simulink model "ICCMA_posicast_23_parallelGCNM_FO"  (R2022b)
settings: Solver=FixedStepAuto  StartTime=0.0  StopTime=1  FixedStep=1e-6  RelTol=1e-3
values from neighbouring files (symbols this model uses):
  alphaFoPar = alpha    [Flyback_SOC_benchmark_Start_parallel.m]
  amp = 1    [Flyback_SOC_benchmark_Start_parallel.m]
  delta = 0.7    [Flyback_SOC_benchmark_Start_parallel.m]
  k1 = 7.51277596604741e-09    (= 7.51277596605e-09)    [Flyback_SOC_benchmark_Start_parallel.m]
  k2 = 1e5    (= 100000)    [Flyback_SOC_benchmark_Start_parallel.m]
  maxKd = 0.1    [Flyback_SOC_benchmark_Start_parallel.m]
  maxKi = 8e5    (= 800000)    [Flyback_SOC_benchmark_Start_parallel.m]
  maxKp = 1e-3    (= 0.001)    [Flyback_SOC_benchmark_Start_parallel.m]
  maxLimDelta = 1.1    [Flyback_SOC_benchmark_Start_parallel.m]
  maxLimTd = 1e-5    (= 1e-05)    [Flyback_SOC_benchmark_Start_parallel.m]
  minKd = 0.001    [Flyback_SOC_benchmark_Start_parallel.m]
  minKi = 8e4    (= 80000)    [Flyback_SOC_benchmark_Start_parallel.m]
  minKp = 1e-6    (= 1e-06)    [Flyback_SOC_benchmark_Start_parallel.m]
  minLimDelta = 0.9    [Flyback_SOC_benchmark_Start_parallel.m]
  minLimTd = 1e-7    (= 1e-07)    [Flyback_SOC_benchmark_Start_parallel.m]
  N = 100    [Flyback_SOC_benchmark_Start_parallel.m]
  optimPeriod = 1/1000    (= 0.001)    [Flyback_SOC_benchmark_Start_parallel.m]
  OVLim = 1    [Flyback_SOC_benchmark_Start_parallel.m]
  refSignalPeriod = 1/1000    (= 0.001)    [Flyback_SOC_benchmark_Start_parallel.m]
  resetThreshold = 0.1    [Flyback_SOC_benchmark_Start_parallel.m]
  td = 24e-6    (= 2.4e-05)    [Flyback_SOC_benchmark_Start_parallel.m]
  TSLim = 65    [Flyback_SOC_benchmark_Start_parallel.m]
libraries: cstblocks x28, dspmathops x7, slpidlib x7
(part 1 of 2)
settings Model: Creator=justu  LastModifiedBy=jairo
settings ModelReferenceCC: EnableRefExpFcnMdlSchedulingChecks=on

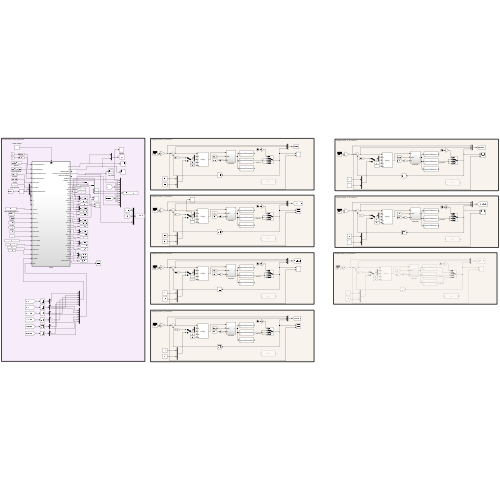
[thumbnail: Simulink's stored preview of the top-level diagram]
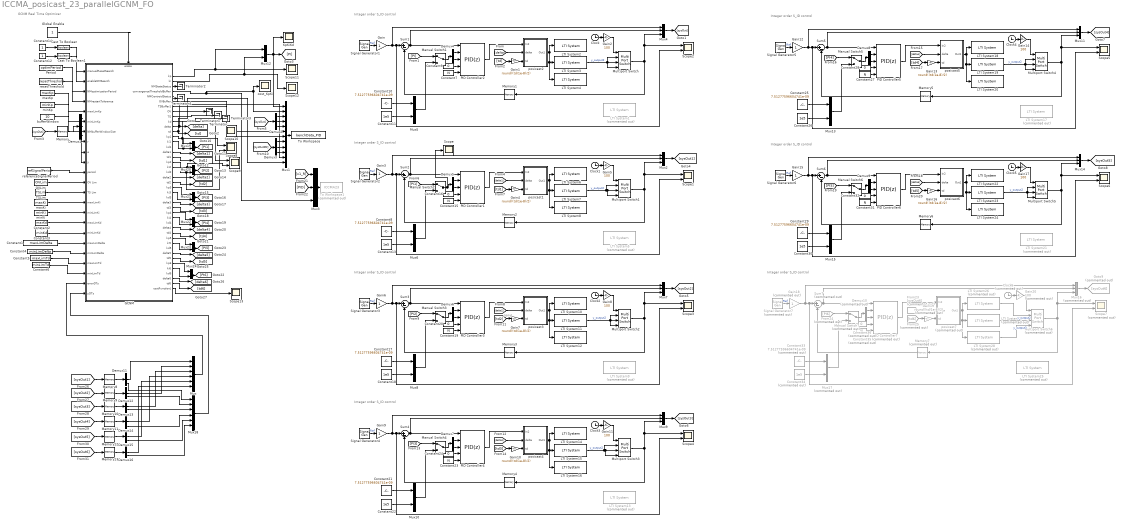
== system ICCMA_posicast_23_parallelGCNM_FO ==
  note: convJ
  note: GCNM Real Time Optimizer
  note: Integer order S_ID control
  note: Integer order S_ID control
  note: Integer order S_ID control
  note: Integer order S_ID control
  note: Integer order S_ID control
  note: Integer order S_ID control
  note: Integer order S_ID control
  Cast To Boolean : DataTypeConversion  OutDataTypeStr=boolean  SaturateOnIntegerOverflow=off  RndMeth=Floor
  Cast To Boolean1 : DataTypeConversion  OutDataTypeStr=boolean  SaturateOnIntegerOverflow=off  RndMeth=Floor
  Clock{,1..5} (6 alike) : Clock
  Clock6 : Clock  Commented=on
  Constant1 : Constant  Value=maxLimDelta
  Constant{8,10,17,21,25,29} (6 alike) : Constant  Value=7.51277596604741e-09
  Constant{11,13,18,22,26,30} (6 alike) : Constant  Value=1e5
  Constant12 : Constant  OutDataTypeStr=boolean
  Constant14 : Constant
  Constant{7,15,19,23,27,31} (6 alike) : Constant  Value=N
  Constant{9,16,20,24,28,32} (6 alike) : Constant  Value=0
  Constant2 : Constant  Value=maxKd
  Constant3 : Constant  Value=minKd
  Constant33 : Constant  Commented=on  Value=7.51277596604741e-09
  Constant34 : Constant  Commented=on  Value=1e5
  Constant35 : Constant  Commented=on  Value=N
  Constant36 : Constant  Commented=on  Value=0
  Constant4 : Constant  Value=minLimDelta
  Constant5 : Constant  Value=maxLimTd
  Constant6 : Constant  Value=minLimTd
  Demux{1..3,11..16} (9 alike) : Demux  Outputs=3
  Demux10 : Demux  Commented=on  Outputs=2
  Demux{4..9} (6 alike) : Demux  Outputs=2
  From23 : From  Commented=on  GotoTag=sysOut6
  From24 : From  Commented=on  GotoTag=PI6
  From25 : From  Commented=on  GotoTag=td6
  GCNM : Subsystem
  Gain{,3,6,9,12,15} (6 alike) : Gain
  Gain{1,4,7,10,13,16} (6 alike) : Gain  Gain=round((td/1e-8)/2)
  Gain{2,5,8,11,14,17} (6 alike) : Gain  Gain=100
  Gain18 : Gain  Commented=on
  Gain19 : Gain  Commented=on  Gain=round((td/1e-8)/2)
  Gain20 : Gain  Commented=on  Gain=100
  Global Enable : Constant
  Goto9 : Goto  Commented=on  GotoTag=sysOut6
  KpKiKd : Scope
  LTI System{1,5,9,13,17,21,25} (7 alike) : cstblocks/LTI System  Commented=on  sys=flybackTFDiscrete  IC=[]
  LTI System{2,6,10,14,18,22} (6 alike) : cstblocks/LTI System  sys=flybackTFDiscrete1  IC=[]
  LTI System{3,7,11,15,19,23} (6 alike) : cstblocks/LTI System  sys=flybackTFDiscrete2  IC=[]
  LTI System{4,8,12,16,20,24} (6 alike) : cstblocks/LTI System  sys=flybackTFDiscrete3  IC=[]
  LTI System26 : cstblocks/LTI System  Commented=on  sys=flybackTFDiscrete1  IC=[]
  LTI System27 : cstblocks/LTI System  Commented=on  sys=flybackTFDiscrete2  IC=[]
  LTI System28 : cstblocks/LTI System  Commented=on  sys=flybackTFDiscrete3  IC=[]
  Manual Switch{1..6} (6 alike) : ManualSwitch
  Manual Switch7 : ManualSwitch  Commented=on
  Memory{,8..13} (7 alike) : Memory  InheritSampleTime=on  LinearizeAsDelay=on
  Memory{1..6} (6 alike) : Memory
  Memory7 : Memory  Commented=on
  Multiport Switch{,1..5} (6 alike) : MultiPortSwitch  DataPortOrder=Specify indices  DataPortIndices={5,10,15}  DiagnosticForDefault=None  SaturateOnIntegerOverflow=off  InputSameDT=off
  Multiport Switch6 : MultiPortSwitch  Commented=on  DataPortOrder=Specify indices  DataPortIndices={5,10,15}  DiagnosticForDefault=None  SaturateOnIntegerOverflow=off  InputSameDT=off
  Mux : Mux  Inputs=6
  Mux1 : Mux  Inputs=12
  Mux{5..6,8,10,12..13,15,19..24} (13 alike) : Mux  Inputs=2
  Mux{2..4,7,9,11,14} (7 alike) : Mux  Inputs=3
  Mux16 : Mux  Commented=on  Inputs=3
  Mux17 : Mux  Commented=on  Inputs=2
  Mux18 : Mux  Inputs=6
  OVLim : Constant  Value=OVLim
  PID Controller{1..6} (6 alike) : slpidlib/PID Controller  Controller=PID  Form=Parallel  TimeDomain=Discrete-time  UseExternalTs=off  SampleTime=-1  IntegratorMethod=Forward Euler  FilterMethod=Forward Euler  ControllerParametersSource=external  P=1  I=100  UseKiTs=off  D=0  N=100  UseFilter=on  TunerSelectOption=Transfer Function Based (PID Tuner App)  InitialConditionSource=internal  InitialConditionForIntegrator=0  InitialConditionForFilter=0  DifferentiatorICPrevScaledInput=0  ExternalReset=none  TrackingMode=off  Kt=1  LimitOutput=off  SatLimitsSource=internal  UpperSaturationLimit=inf  LowerSaturationLimit=-inf  LinearizeAsGain=on  AntiWindupMode=none  Kb=1  LimitIntegrator=off  UpperIntegratorSaturationLimit=inf  LowerIntegratorSaturationLimit=-inf  POutMin=[]  POutMax=[]  IOutMin=[]  IOutMax=[]  DOutMin=[]  DOutMax=[]  NOutMin=[]  NOutMax=[]  SumOutMin=[]  SumOutMax=[]  SaturationOutMin=[]  SaturationOutMax=[]  PParamMin=[]  PParamMax=[]  IParamMin=[]  IParamMax=[]  DParamMin=[]  DParamMax=[]  NParamMin=[]  NParamMax=[]  KbParamMin=[]  KbParamMax=[]  KtParamMin=[]  KtParamMax=[]  KbOutMin=[]  KbOutMax=[]  KtOutMin=[]  KtOutMax=[]  IntegratorOutMin=[]  IntegratorOutMax=[]  FilterOutMin=[]  FilterOutMax=[]  SumI1OutMin=[]  SumI1OutMax=[]  SumI2OutMin=[]  SumI2OutMax=[]  SumI3OutMin=[]  SumI3OutMax=[]  SumI4OutMin=[]  SumI4OutMax=[]  SumDOutMin=[]  SumDOutMax=[]  DifferentiatorOutMin=[]  DifferentiatorOutMax=[]  FilterDiffOutCoefMin=[]  FilterDiffOutCoefMax=[]  ReciprocalOutMin=[]  ReciprocalOutMax=[]  SumDenOutMin=[]  SumDenOutMax=[]  SumNumOutMin=[]  SumNumOutMax=[]  DivideOutMin=[]  DivideOutMax=[]  UdiffTsProdOutMin=[]  UdiffTsProdOutMax=[]  NTsProdOutMin=[]  NTsProdOutMax=[]  UintegralTsProdOutMin=[]  UintegralTsProdOutMax=[]  UngainTsProdOutMin=[]  UngainTsProdOutMax=[]  ClampingZeroOutDataTypeStr=Inherit: Inherit via back propagation  ClampingZeroOutMin=[]  ClampingZeroOutMax=[]  FilterDenConstantOutDataTypeStr=Inherit: Inherit via back propagation  FilterDenConstantOutMin=[]  FilterDenConstantOutMax=[]  PCopyOutDataTypeStr=Inherit: Inherit via back propagation  PCopyOutMin=[]  PCopyOutMax=[]  NCopyOutDataTypeStr=Inherit: Inherit via back propagation  NCopyOutMin=[]  NCopyOutMax=[]  IntegratorContinuousStateAttributes=''  IntegratorStateMustResolveToSignalObject=off  IntegratorRTWStateStorageClass=Auto  FilterContinuousStateAttributes=''  FilterStateMustResolveToSignalObject=off  FilterRTWStateStorageClass=Auto  ParallelPVariant=ExternalParameters  IdealPVariant=Disabled  IVariant=ExternalParameters  DVariant=ExternalParameters  IntegratorVariant=Discrete  SatVariant=Disabled  AWVariant=Passthrough  PCopyVariant=Disabled  TRVariant=Disabled  FdbkBlocksVariant=Forward  IdealPFdbkVariant=Disabled  SatFdbkVariant=Disabled  DerivativeFilterVariant=ForwardEulerFilter  NVariant=ExternalParameters  NCopyVariant=Disabled  FilterICVariant=InternalICsFilter  IntegratorICVariant=InternalICs  ExternalResetVariant=Disabled  TRSumVariant=Passthrough  SumFdbkVariant=Disabled  SumVariant=Sum_PID  TsampFilterVariant=InternalTs  TsampNgainVariant=Passthrough  TsampIntegralVariant=Passthrough  ExternalSaturationOutDataTypeStr=Inherit: Same as second input
  PID Controller7 : slpidlib/PID Controller  Commented=on  Controller=PID  Form=Parallel  TimeDomain=Discrete-time  UseExternalTs=off  SampleTime=-1  IntegratorMethod=Forward Euler  FilterMethod=Forward Euler  ControllerParametersSource=external  P=1  I=100  UseKiTs=off  D=0  N=100  UseFilter=on  TunerSelectOption=Transfer Function Based (PID Tuner App)  InitialConditionSource=internal  InitialConditionForIntegrator=0  InitialConditionForFilter=0  DifferentiatorICPrevScaledInput=0  ExternalReset=none  TrackingMode=off  Kt=1  LimitOutput=off  SatLimitsSource=internal  UpperSaturationLimit=inf  LowerSaturationLimit=-inf  LinearizeAsGain=on  AntiWindupMode=none  Kb=1  LimitIntegrator=off  UpperIntegratorSaturationLimit=inf  LowerIntegratorSaturationLimit=-inf  POutMin=[]  POutMax=[]  IOutMin=[]  IOutMax=[]  DOutMin=[]  DOutMax=[]  NOutMin=[]  NOutMax=[]  SumOutMin=[]  SumOutMax=[]  SaturationOutMin=[]  SaturationOutMax=[]  PParamMin=[]  PParamMax=[]  IParamMin=[]  IParamMax=[]  DParamMin=[]  DParamMax=[]  NParamMin=[]  NParamMax=[]  KbParamMin=[]  KbParamMax=[]  KtParamMin=[]  KtParamMax=[]  KbOutMin=[]  KbOutMax=[]  KtOutMin=[]  KtOutMax=[]  IntegratorOutMin=[]  IntegratorOutMax=[]  FilterOutMin=[]  FilterOutMax=[]  SumI1OutMin=[]  SumI1OutMax=[]  SumI2OutMin=[]  SumI2OutMax=[]  SumI3OutMin=[]  SumI3OutMax=[]  SumI4OutMin=[]  SumI4OutMax=[]  SumDOutMin=[]  SumDOutMax=[]  DifferentiatorOutMin=[]  DifferentiatorOutMax=[]  FilterDiffOutCoefMin=[]  FilterDiffOutCoefMax=[]  ReciprocalOutMin=[]  ReciprocalOutMax=[]  SumDenOutMin=[]  SumDenOutMax=[]  SumNumOutMin=[]  SumNumOutMax=[]  DivideOutMin=[]  DivideOutMax=[]  UdiffTsProdOutMin=[]  UdiffTsProdOutMax=[]  NTsProdOutMin=[]  NTsProdOutMax=[]  UintegralTsProdOutMin=[]  UintegralTsProdOutMax=[]  UngainTsProdOutMin=[]  UngainTsProdOutMax=[]  ClampingZeroOutDataTypeStr=Inherit: Inherit via back propagation  ClampingZeroOutMin=[]  ClampingZeroOutMax=[]  FilterDenConstantOutDataTypeStr=Inherit: Inherit via back propagation  FilterDenConstantOutMin=[]  FilterDenConstantOutMax=[]  PCopyOutDataTypeStr=Inherit: Inherit via back propagation  PCopyOutMin=[]  PCopyOutMax=[]  NCopyOutDataTypeStr=Inherit: Inherit via back propagation  NCopyOutMin=[]  NCopyOutMax=[]  IntegratorContinuousStateAttributes=''  IntegratorStateMustResolveToSignalObject=off  IntegratorRTWStateStorageClass=Auto  FilterContinuousStateAttributes=''  FilterStateMustResolveToSignalObject=off  FilterRTWStateStorageClass=Auto  ParallelPVariant=ExternalParameters  IdealPVariant=Disabled  IVariant=ExternalParameters  DVariant=ExternalParameters  IntegratorVariant=Discrete  SatVariant=Disabled  AWVariant=Passthrough  PCopyVariant=Disabled  TRVariant=Disabled  FdbkBlocksVariant=Forward  IdealPFdbkVariant=Disabled  SatFdbkVariant=Disabled  DerivativeFilterVariant=ForwardEulerFilter  NVariant=ExternalParameters  NCopyVariant=Disabled  FilterICVariant=InternalICsFilter  IntegratorICVariant=InternalICs  ExternalResetVariant=Disabled  TRSumVariant=Passthrough  SumFdbkVariant=Disabled  SumVariant=Sum_PID  TsampFilterVariant=InternalTs  TsampNgainVariant=Passthrough  TsampIntegralVariant=Passthrough  ExternalSaturationOutDataTypeStr=Inherit: Same as second input
  Period : Constant  Value=optimPeriod  OutDataTypeStr=double
  Scope{,11..13} (4 alike) : Scope
  Scope{1..6,8..10} (9 alike) : Scope  NumInputPorts=2
  Scope7 : Scope  Commented=on  NumInputPorts=2
  Signal Generator{1..6} (6 alike) : SignalGenerator  WaveForm=square  Frequency=1000
  Signal Generator7 : SignalGenerator  Commented=on  WaveForm=square  Frequency=1000
  Sum{1..6} (6 alike) : Sum  Inputs=|+-
  Sum7 : Sum  Commented=on  Inputs=|+-
  TSLim : Constant  Value=TSLim
  Terminator{,1..4} (5 alike) : Terminator
  To Workspace : ToWorkspace  VariableName=benchData_PID  SaveFormat=Timeseries  SampleTime=-1
  To Workspace1 : ToWorkspace  Commented=on  VariableName=ICCMA23  SaveFormat=Timeseries  SampleTime=-1
  bufferWindow : Constant  Value=10  OutDataTypeStr=uint16
  cost_KpKi : Scope
  maxKi : Constant  Value=maxKi  VectorParams1D=off  OutDataTypeStr=double
  maxKp : Constant  Value=maxKp  OutDataTypeStr=double
  minKi : Constant  Value=minKi  OutDataTypeStr=double
  minKp : Constant  Value=minKp  OutDataTypeStr=double
  posicast1 : Subsystem
  posicast2 : Subsystem
  posicast3 : Subsystem
  posicast4 : Subsystem
  posicast5 : Subsystem
  posicast6 : Subsystem
  posicast7 : Subsystem  Commented=on
  referenceSignalPeriod : Constant  Value=refSignalPeriod
  resetThreshold : Constant  Value=resetThreshold
  wires:
  Gain/1 -> Scope2/2, Sum1/1, Mux4/1
  Mux5/1 -> Manual Switch1/2
  Memory/1 -> Demux1/1
  TSLim/1 -> GCNM/13(TS Lim)
  Constant9/1 -> PID Controller2/4
  Demux1/1 -> GCNM/8("  r")
  [PI] -> Manual Switch1/1
  PID Controller2/1 -> posicast2/1(In2)
  referenceSignalPeriod/1 -> GCNM/11("  period")
  Constant14/1 -> Cast To Boolean/1
  Manual Switch1/1 -> Demux4/1
  Demux2/1 -> Mux1/3
  Mux1/1 -> To Workspace/1
  Sum1/1 -> Mux4/2, PID Controller2/1
  Mux3/1 -> To Workspace1/1
  bufferWindow/1 -> GCNM/7(NMbufferWindowSize)
  Constant12/1 -> Cast To Boolean1/1
  [sysOut] -> Demux2/1
  GCNM/2("  ki") -> Scope12/1, Mux12/2
  resetThreshold/1 -> GCNM/4(NMrestartTolerance)
  Constant7/1 -> PID Controller2/5
  Demux3/1 -> Mux1/8
  GCNM/9(TS) -> Terminator/1
  Cast To Boolean/1 -> GCNM/1(manualResetSearch)
  Cast To Boolean1/1 -> GCNM/2(enableNMSearch)
  Demux1/3 -> GCNM/10("  y")
  Demux2/3 -> Mux1/5
  [PID] -> Mux3/2
  GCNM/1("  kp") -> Scope11/1, Mux12/1
  Demux2/2 -> Mux1/4
  [x1_R] -> Mux3/1
  Mux4/1 -> [sysOut]
  GCNM/5(NMCentroidStatus) -> Terminator4/1
  Global Enable/1 -> GCNM/Enable
  Demux1/2 -> GCNM/9("  e")
  Demux4/2 -> PID Controller2/3
  GCNM/10(kd) -> Terminator3/1
  GCNM/7(TSBuffer1) -> Mux1/7
  Demux4/1 -> PID Controller2/2
  Mux12/1 -> Mux1/1, KpKiKd/1, [PI]
  maxKi/1 -> GCNM/14(maxLimKi)
  maxKp/1 -> GCNM/5(maxLimKp)
  Period/1 -> GCNM/3(NMoptimizationPeriod)
  Signal Generator1/1 -> Gain/1  "Ref"
  GCNM/6(OVBuffer) -> Mux1/6
  GCNM/4(convergenceThresholdBuffer) -> Mux1/2, cost_KpKi/1, Mux3/3
  Constant10/1 -> Mux5/1
  Constant2/1 -> GCNM/16(maxLimKd)
  Demux3/2 -> Mux1/9
  Constant11/1 -> Mux5/2
  Constant3/1 -> GCNM/17(minLimKd)
  minKi/1 -> GCNM/15(minLimKi)
  [sysOut] -> Memory/1
  minKp/1 -> GCNM/6(minLimKp)
  [sysOutZN] -> Demux3/1
  OVLim/1 -> GCNM/12("  OV Lim")
  GCNM/3(NMStateStatus) -> Terminator2/1
  GCNM/8(OV) -> Terminator1/1
  Demux3/3 -> Mux1/10
  posicast2/1(Out1) -> LTI System4/1, LTI System3/1, LTI System2/1
  GCNM/11(delta) -> Mux1/11, [delta]
  GCNM/12(td) -> [td], Mux1/12
  [td] -> Gain1/1
  Gain1/1 -> posicast2/3(td)
  [delta] -> posicast2/2(delta)
  Constant1/1 -> GCNM/18(maxLimDelta)
  Constant4/1 -> GCNM/19(minLimDelta)
  Constant5/1 -> GCNM/20(maxLimTd)
  Constant6/1 -> GCNM/21(minLimTd)
  Clock/1 -> Gain2/1
  Multiport Switch/1 -> Memory1/1, Mux4/3, Scope2/1
  Gain2/1 -> Multiport Switch/1
  Memory1/1 -> Sum1/2
  LTI System3/1 -> Multiport Switch/2, Multiport Switch/4, Multiport Switch/3  "y_output2"
  LTI System7/1 -> Multiport Switch1/2, Multiport Switch1/4, Multiport Switch1/3  "y_output2"
  Memory2/1 -> Sum2/2
  Gain5/1 -> Multiport Switch1/1
  PID Controller1/1 -> posicast1/1(In2)
  Multiport Switch1/1 -> Memory2/1, Mux2/3, Scope1/1
  Constant13/1 -> Mux6/2
  [td1] -> Gain4/1
  posicast1/1(Out1) -> LTI System8/1, LTI System7/1, LTI System6/1
  [delta1] -> posicast1/2(delta)
  Constant15/1 -> PID Controller1/5
  Signal Generator2/1 -> Gain3/1  "Ref"
  Clock1/1 -> Gain5/1
  Constant8/1 -> Mux6/1
  Mux2/1 -> [sysOut1]
  Sum2/1 -> Mux2/2, PID Controller1/1
  Demux5/1 -> PID Controller1/2
  Demux5/2 -> PID Controller1/3
  Constant16/1 -> PID Controller1/4
  Manual Switch2/1 -> Scope/1, Demux5/1
  Gain3/1 -> Scope1/2, Sum2/1, Mux2/1
  [PI1] -> Manual Switch2/1
  Gain4/1 -> posicast1/3(td)
  Mux6/1 -> Manual Switch2/2
  LTI System11/1 -> Multiport Switch2/4, Multiport Switch2/2, Multiport Switch2/3  "y_output2"
  Memory3/1 -> Sum3/2
  Gain8/1 -> Multiport Switch2/1
  PID Controller3/1 -> posicast3/1(In2)
  Multiport Switch2/1 -> Memory3/1, Mux7/3, Scope3/1
  Constant18/1 -> Mux8/2
  [td2] -> Gain7/1
  posicast3/1(Out1) -> LTI System12/1, LTI System11/1, LTI System10/1
  [delta2] -> posicast3/2(delta)
  Constant19/1 -> PID Controller3/5
  Signal Generator3/1 -> Gain6/1  "Ref"
  Clock2/1 -> Gain8/1
  Constant17/1 -> Mux8/1
  Mux7/1 -> [sysOut2]
  Sum3/1 -> Mux7/2, PID Controller3/1
  Demux6/1 -> PID Controller3/2
  Demux6/2 -> PID Controller3/3
  Constant20/1 -> PID Controller3/4
  Manual Switch3/1 -> Demux6/1
  Gain6/1 -> Scope3/2, Sum3/1, Mux7/1
  [PI2] -> Manual Switch3/1
  Gain7/1 -> posicast3/3(td)
  Mux8/1 -> Manual Switch3/2
  LTI System15/1 -> Multiport Switch3/2, Multiport Switch3/4, Multiport Switch3/3  "y_output2"
  Memory4/1 -> Sum4/2
  Gain11/1 -> Multiport Switch3/1
  PID Controller4/1 -> posicast4/1(In2)
  Multiport Switch3/1 -> Memory4/1, Mux9/3, Scope4/1
  Constant22/1 -> Mux10/2
  [td3] -> Gain10/1
  posicast4/1(Out1) -> LTI System16/1, LTI System15/1, LTI System14/1
  [delta3] -> posicast4/2(delta)
  Constant23/1 -> PID Controller4/5
  Signal Generator4/1 -> Gain9/1  "Ref"
  Clock3/1 -> Gain11/1
  Constant21/1 -> Mux10/1
  Mux9/1 -> [sysOut3]
  Sum4/1 -> Mux9/2, PID Controller4/1
  Demux7/1 -> PID Controller4/2
  Demux7/2 -> PID Controller4/3
  Constant24/1 -> PID Controller4/4
  Manual Switch4/1 -> Demux7/1
  Gain9/1 -> Scope4/2, Sum4/1, Mux9/1
  [PI3] -> Manual Switch4/1
  Gain10/1 -> posicast4/3(td)
  Mux10/1 -> Manual Switch4/2
  LTI System19/1 -> Multiport Switch4/2, Multiport Switch4/4, Multiport Switch4/3  "y_output2"
  Memory5/1 -> Sum5/2
  Gain14/1 -> Multiport Switch4/1
  PID Controller5/1 -> posicast5/1(In2)
  Multiport Switch4/1 -> Memory5/1, Mux11/3, Scope5/1
  Constant26/1 -> Mux13/2
  [td4] -> Gain13/1
  posicast5/1(Out1) -> LTI System20/1, LTI System19/1, LTI System18/1
  [delta4] -> posicast5/2(delta)
  Constant27/1 -> PID Controller5/5
  Signal Generator5/1 -> Gain12/1  "Ref"
  Clock4/1 -> Gain14/1
  Constant25/1 -> Mux13/1
  Mux11/1 -> [sysOut4]
  Sum5/1 -> Mux11/2, PID Controller5/1
  Demux8/1 -> PID Controller5/2
  Demux8/2 -> PID Controller5/3
  Constant28/1 -> PID Controller5/4
  Manual Switch5/1 -> Demux8/1
  Gain12/1 -> Scope5/2, Sum5/1, Mux11/1
  [PI4] -> Manual Switch5/1
  Gain13/1 -> posicast5/3(td)
  Mux13/1 -> Manual Switch5/2
  LTI System23/1 -> Multiport Switch5/2, Multiport Switch5/4, Multiport Switch5/3  "y_output2"
  Memory6/1 -> Sum6/2
  Gain17/1 -> Multiport Switch5/1
  PID Controller6/1 -> posicast6/1(In2)
  Multiport Switch5/1 -> Memory6/1, Mux14/3, Scope6/1
  Constant30/1 -> Mux15/2
  [td5] -> Gain16/1
  posicast6/1(Out1) -> LTI System24/1, LTI System23/1, LTI System22/1
  [delta5] -> posicast6/2(delta)
  Constant31/1 -> PID Controller6/5
  Signal Generator6/1 -> Gain15/1  "Ref"
  Clock5/1 -> Gain17/1
  Constant29/1 -> Mux15/1
  Mux14/1 -> [sysOut5]
  Sum6/1 -> Mux14/2, PID Controller6/1
  Demux9/1 -> PID Controller6/2
  Demux9/2 -> PID Controller6/3
  Constant32/1 -> PID Controller6/4
  Manual Switch6/1 -> Demux9/1
  Gain15/1 -> Scope6/2, Sum6/1, Mux14/1
  [PI5] -> Manual Switch6/1
  Gain16/1 -> posicast6/3(td)
  Mux15/1 -> Manual Switch6/2
  LTI System27/1 -> Multiport Switch6/3  "y_output2"
  Memory7/1 -> Sum7/2
  Gain20/1 -> Multiport Switch6/1
  PID Controller7/1 -> posicast7/1(In2)
  Multiport Switch6/1 -> Memory7/1, Mux16/3, Scope7/1
  Constant34/1 -> Mux17/2
  LTI System26/1 -> Multiport Switch6/2
  From25/1 -> Gain19/1
  posicast7/1(Out1) -> LTI System28/1, LTI System27/1, LTI System26/1
  From23/1 -> posicast7/2(delta)
  Constant35/1 -> PID Controller7/5
  Signal Generator7/1 -> Gain18/1  "Ref"
  Clock6/1 -> Gain20/1
  Constant33/1 -> Mux17/1
  Mux16/1 -> Goto9/1
  Sum7/1 -> Mux16/2, PID Controller7/1
  Demux10/1 -> PID Controller7/2
  Demux10/2 -> PID Controller7/3
  Constant36/1 -> PID Controller7/4
  LTI System28/1 -> Multiport Switch6/4  "y_output3"
  Manual Switch7/1 -> Demux10/1
  Gain18/1 -> Scope7/2, Sum7/1, Mux16/1
  From24/1 -> Manual Switch7/1
  Gain19/1 -> posicast7/3(td)
  Mux17/1 -> Manual Switch7/2
  [sysOut1] -> Memory8/1
  Memory8/1 -> Demux11/1
  Demux11/2 -> Mux/1
  Memory9/1 -> Demux12/1
  Demux12/2 -> Mux/2
  [sysOut2] -> Memory9/1
  [sysOut3] -> Memory10/1
  Demux13/2 -> Mux/3
  Memory10/1 -> Demux13/1
  [sysOut4] -> Memory11/1
  Demux14/2 -> Mux/4
  Memory11/1 -> Demux14/1
  [sysOut5] -> Memory12/1
  Demux15/2 -> Mux/5
  Memory12/1 -> Demux15/1
  [sysOut6] -> Memory13/1
  Demux16/2 -> Mux/6
  Memory13/1 -> Demux16/1
  Demux11/3 -> Mux18/1
  Demux13/3 -> Mux18/3
  Demux14/3 -> Mux18/4
  Demux15/3 -> Mux18/5
  Demux16/3 -> Mux18/6
  Demux12/3 -> Mux18/2
  Mux/1 -> GCNM/22(errorDTs)
  Mux18/1 -> GCNM/23(yDTs)
  Mux19/1 -> [PI1]
  GCNM/16(delta1) -> [delta1]
  GCNM/17(td1) -> [td1]
  GCNM/13("  kp1") -> Mux19/1, Scope9/1
  GCNM/22(td2) -> [td2]
  Mux20/1 -> [PI2]
  GCNM/21(delta2) -> [delta2]
  GCNM/19("  ki2") -> Scope8/2, Mux20/2
  GCNM/18("  kp2") -> Scope9/2, Mux20/1
  GCNM/27(td3) -> [td3]
  Mux21/1 -> [PI3]
  GCNM/26(delta3) -> [delta3]
  GCNM/24("  ki3") -> Mux21/2
  GCNM/23("  kp3") -> Mux21/1
  GCNM/29("  ki4") -> Mux22/2
  GCNM/31(delta4) -> [delta4]
  GCNM/32(td4) -> [td4]
  GCNM/28("  kp4") -> Mux22/1
  Mux22/1 -> [PI4]
  GCNM/36(delta5) -> [delta5]
  GCNM/33("  kp5") -> Mux23/1
  Mux23/1 -> [PI5]
  GCNM/34("  ki5") -> Mux23/2
  GCNM/37(td5) -> [td5]
  Mux24/1 -> [PI6]
  GCNM/41(delta6) -> [delta6]
  GCNM/42(td6) -> [td6]
  GCNM/38("  kp6") -> Mux24/1
  GCNM/39("  ki6") -> Mux24/2
  GCNM/14("  ki1") -> Scope8/1, Mux19/2
  GCNM/43(costFunctionJ) -> Scope13/1

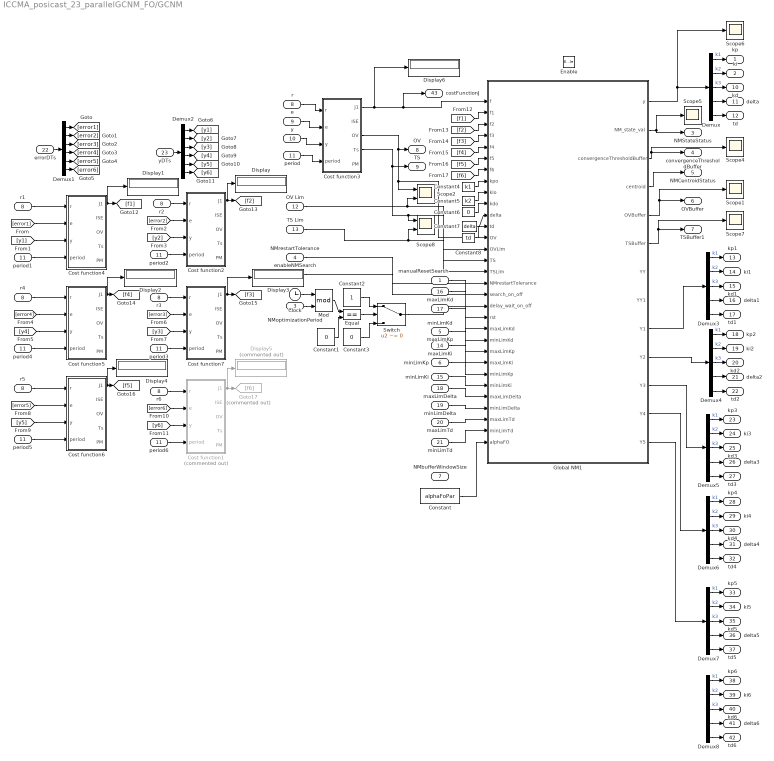
== system ICCMA_posicast_23_parallelGCNM_FO/GCNM ==
  manualResetSearch : Inport  OutDataTypeStr=boolean
  enableNMSearch : Inport  Port=2  OutDataTypeStr=boolean
  NMoptimizationPeriod : Inport  Port=3  OutDataTypeStr=double
  NMrestartTolerance : Inport  Port=4
  maxLimKp : Inport  Port=5  OutDataTypeStr=double
  minLimKp : Inport  Port=6  OutDataTypeStr=double
  NMbufferWindowSize : Inport  Port=7  OutDataTypeStr=uint16
  "  r" : Inport  Port=8  OutDataTypeStr=double
  "  e" : Inport  Port=9  OutDataTypeStr=double
  "  y" : Inport  Port=10  OutDataTypeStr=double
  "  period" : Inport  Port=11  OutDataTypeStr=double
  "  OV Lim" : Inport  Port=12  OutDataTypeStr=double
  TS Lim : Inport  Port=13  OutDataTypeStr=double
  maxLimKi : Inport  Port=14  OutDataTypeStr=double
  minLimKi : Inport  Port=15  OutDataTypeStr=double
  maxLimKd : Inport  Port=16
  minLimKd : Inport  Port=17
  maxLimDelta : Inport  Port=18
  minLimDelta : Inport  Port=19
  maxLimTd : Inport  Port=20
  minLimTd : Inport  Port=21
  errorDTs : Inport  Port=22
  yDTs : Inport  Port=23
  Enable : EnablePort
    period{1..6} (6 alike) : InportShadow  Port=11  OutDataTypeStr=double
    r{1..6} (6 alike) : InportShadow  Port=8  OutDataTypeStr=double
  Clock : Clock
  Constant : Constant  Value=alphaFoPar
  Constant1 : Constant  Value=0
  Constant2 : Constant
  Constant3 : Constant  Value=0
  Constant4 : Constant  Value=k1
  Constant5 : Constant  Value=k2
  Constant6 : Constant  Value=0
  Constant7 : Constant  Value=delta
  Constant8 : Constant  Value=td
  Cost function1 : Subsystem  Commented=on
  Cost function2 : Subsystem
  Cost function3 : Subsystem
  Cost function4 : Subsystem
  Cost function5 : Subsystem
  Cost function6 : Subsystem
  Cost function7 : Subsystem
  Demux{,3..8} (7 alike) : Demux  Outputs=5
  Demux1 : Demux  Outputs=6
  Demux2 : Demux  Outputs=6
  Display{,1..4,6} (6 alike) : Display
  Display5 : Display  Commented=on
  Equal : RelationalOperator  Operator===  RndMeth=Simplest  InputSameDT=off
  Global NM1 : MATLAB Function  TreatAsAtomicUnit=on
  Goto17 : Goto  Commented=on  GotoTag=f6
  Mod : Math  Operator=mod
  Scope{1,4..7} (5 alike) : Scope
  Scope2 : Scope  NumInputPorts=2
  Scope8 : Scope  NumInputPorts=2
  Switch : Switch  Criteria=u2 ~= 0  SaturateOnIntegerOverflow=off  InputSameDT=off
  "  kp" : Outport  OutDataTypeStr=double
  "  ki" : Outport  Port=2  OutDataTypeStr=double
  NMStateStatus : Outport  Port=3  OutDataTypeStr=double
  convergenceThresholdBuffer : Outport  Port=4  OutDataTypeStr=double
  NMCentroidStatus : Outport  Port=5  OutDataTypeStr=double
  OVBuffer : Outport  Port=6  OutDataTypeStr=double
  TSBuffer1 : Outport  Port=7  OutDataTypeStr=double
  OV : Outport  Port=8  OutDataTypeStr=double
  TS : Outport  Port=9  OutDataTypeStr=double
  kd : Outport  Port=10
  delta : Outport  Port=11
  td : Outport  Port=12
  "  kp1" : Outport  Port=13  OutDataTypeStr=double
  "  ki1" : Outport  Port=14  OutDataTypeStr=double
  kd1 : Outport  Port=15
  delta1 : Outport  Port=16
  td1 : Outport  Port=17
  "  kp2" : Outport  Port=18  OutDataTypeStr=double
  "  ki2" : Outport  Port=19  OutDataTypeStr=double
  kd2 : Outport  Port=20
  delta2 : Outport  Port=21
  td2 : Outport  Port=22
  "  kp3" : Outport  Port=23  OutDataTypeStr=double
  "  ki3" : Outport  Port=24  OutDataTypeStr=double
  kd3 : Outport  Port=25
  delta3 : Outport  Port=26
  td3 : Outport  Port=27
  "  kp4" : Outport  Port=28  OutDataTypeStr=double
  "  ki4" : Outport  Port=29  OutDataTypeStr=double
  kd4 : Outport  Port=30
  delta4 : Outport  Port=31
  td4 : Outport  Port=32
  "  kp5" : Outport  Port=33  OutDataTypeStr=double
  "  ki5" : Outport  Port=34  OutDataTypeStr=double
  kd5 : Outport  Port=35
  delta5 : Outport  Port=36
  td5 : Outport  Port=37
  "  kp6" : Outport  Port=38  OutDataTypeStr=double
  "  ki6" : Outport  Port=39  OutDataTypeStr=double
  kd6 : Outport  Port=40
  delta6 : Outport  Port=41
  td6 : Outport  Port=42
  costFunctionJ : Outport  Port=43  OutDataTypeStr=double
  wires:
  NMrestartTolerance/1 -> Global NM1/17(NMrestartTolerance)
  manualResetSearch/1 -> Global NM1/20(rst)
  enableNMSearch/1 -> Global NM1/18(search_on_off)
  minLimKp/1 -> Global NM1/25(minLimKp)
  maxLimKp/1 -> Global NM1/23(maxLimKp)
  Global NM1/2(NM_state_val) -> Scope5/1, NMStateStatus/1
  Global NM1/3(convergenceThresholdBuffer) -> Scope4/1, convergenceThresholdBuffer/1
  Global NM1/4(centroid) -> NMCentroidStatus/1
  Global NM1/1(y) -> Demux/1, Scope6/1
  Constant5/1 -> Global NM1/9(kio)
  Cost function3/3(OV) -> OV/1, Scope2/1, Global NM1/13(OV)
  "  y"/1 -> Cost function3/3(y)
  "  e"/1 -> Cost function3/2(e)
  "  r"/1 -> Cost function3/1(r)
  Global NM1/5(OVBuffer) -> Scope1/1, OVBuffer/1
  "  period"/1 -> Cost function3/4(period)
  "  OV Lim"/1 -> Scope2/2, Global NM1/14(OVLim)
  Cost function3/4(Ts) -> TS/1, Global NM1/15(TS), Scope8/1
  TS Lim/1 -> Scope8/2, Global NM1/16(TSLim)
  Global NM1/6(TSBuffer) -> Scope7/1, TSBuffer1/1
  Cost function3/1(J1) -> Display6/1, costFunctionJ/1, Global NM1/1(f)
  Clock/1 -> Mod/1
  NMoptimizationPeriod/1 -> Mod/2
  Constant1/1 -> Equal/2
  Mod/1 -> Equal/1
  Constant2/1 -> Switch/1
  Constant3/1 -> Switch/3
  Switch/1 -> Global NM1/19(delay_wait_on_off)
  Equal/1 -> Switch/2
  maxLimKi/1 -> Global NM1/24(maxLimKi)
  minLimKi/1 -> Global NM1/26(minLimKi)
  maxLimKd/1 -> Global NM1/21(maxLimKd)
  minLimKd/1 -> Global NM1/22(minLimKd)
  Constant6/1 -> Global NM1/10(kdo)
  Constant4/1 -> Global NM1/8(kpo)
  Demux/1 -> "  kp"/1  "k1"
  Demux/3 -> kd/1  "k3"
  Demux/2 -> "  ki"/1  "k2"
  Constant7/1 -> Global NM1/11(delta)
  Constant8/1 -> Global NM1/12(td)
  Demux/5 -> td/1
  Demux/4 -> delta/1
  maxLimDelta/1 -> Global NM1/27(maxLimDelta)
  minLimDelta/1 -> Global NM1/28(minLimDelta)
  maxLimTd/1 -> Global NM1/29(maxLimTd)
  minLimTd/1 -> Global NM1/30(minLimTd)
  errorDTs/1 -> Demux1/1
  Demux1/1 -> [error1]
  Demux1/2 -> [error2]
  Demux1/3 -> [error3]
  Demux1/4 -> [error4]
  Demux1/5 -> [error5]
  Demux1/6 -> [error6]
  Demux2/2 -> [y2]
  Demux2/5 -> [y5]
  Demux2/1 -> [y1]
  Demux2/4 -> [y4]
  Demux2/6 -> [y6]
  Demux2/3 -> [y3]
  yDTs/1 -> Demux2/1
  "  r1"/1 -> Cost function4/1(r)
  "  r2"/1 -> Cost function2/1(r)
  "  r3"/1 -> Cost function7/1(r)
  "  r4"/1 -> Cost function5/1(r)
  "  r5"/1 -> Cost function6/1(r)
  "  r6"/1 -> Cost function1/1(r)
  [error1] -> Cost function4/2(e)
  [y1] -> Cost function4/3(y)
  "  period1"/1 -> Cost function4/4(period)
  "  period2"/1 -> Cost function2/4(period)
  "  period3"/1 -> Cost function7/4(period)
  "  period4"/1 -> Cost function5/4(period)
  "  period5"/1 -> Cost function6/4(period)
  "  period6"/1 -> Cost function1/4(period)
  [error2] -> Cost function2/2(e)
  [y2] -> Cost function2/3(y)
  [error4] -> Cost function5/2(e)
  [y4] -> Cost function5/3(y)
  [y3] -> Cost function7/3(y)
  [error3] -> Cost function7/2(e)
  [error5] -> Cost function6/2(e)
  [y5] -> Cost function6/3(y)
  [y6] -> Cost function1/3(y)
  [error6] -> Cost function1/2(e)
  Cost function4/1(J1) -> Display1/1, [f1]
  Cost function2/1(J1) -> Display/1, [f2]
  Cost function5/1(J1) -> Display2/1, [f4]
  Cost function7/1(J1) -> Display3/1, [f3]
  Cost function6/1(J1) -> Display4/1, [f5]
  Cost function1/1(J1) -> Display5/1, Goto17/1
  [f1] -> Global NM1/2(f1)
  [f2] -> Global NM1/3(f2)
  [f3] -> Global NM1/4(f3)
  [f4] -> Global NM1/5(f4)
  [f5] -> Global NM1/6(f5)
  [f6] -> Global NM1/7(f6)
  Demux3/4 -> delta1/1
  Demux3/5 -> td1/1
  Demux3/2 -> "  ki1"/1  "k2"
  Demux3/3 -> kd1/1  "k3"
  Demux3/1 -> "  kp1"/1  "k1"
  Global NM1/10(Y2) -> Demux4/1
  Demux4/1 -> "  kp2"/1  "k1"
  Demux4/3 -> kd2/1  "k3"
  Demux4/2 -> "  ki2"/1  "k2"
  Demux4/5 -> td2/1
  Demux4/4 -> delta2/1
  Global NM1/9(Y1) -> Demux3/1
  Demux5/4 -> delta3/1
  Demux5/5 -> td3/1
  Demux5/2 -> "  ki3"/1  "k2"
  Demux5/3 -> kd3/1  "k3"
  Demux5/1 -> "  kp3"/1  "k1"
  Global NM1/11(Y3) -> Demux5/1
  Demux6/1 -> "  kp4"/1  "k1"
  Demux6/4 -> delta4/1
  Demux6/3 -> kd4/1  "k3"
  Demux6/2 -> "  ki4"/1  "k2"
  Global NM1/12(Y4) -> Demux6/1
  Demux6/5 -> td4/1
  Demux7/1 -> "  kp5"/1  "k1"
  Demux7/4 -> delta5/1
  Demux7/3 -> kd5/1  "k3"
  Demux7/2 -> "  ki5"/1  "k2"
  Global NM1/13(Y5) -> Demux7/1
  Demux7/5 -> td5/1
  Demux8/1 -> "  kp6"/1  "k1"
  Demux8/4 -> delta6/1
  Demux8/3 -> kd6/1  "k3"
  Demux8/2 -> "  ki6"/1  "k2"
  Demux8/5 -> td6/1
  Constant/1 -> Global NM1/31(alphaFO)

== system ICCMA_posicast_23_parallelGCNM_FO/posicast1 ==
  In2 : Inport
  delta : Inport  Port=2
  td : Inport  Port=3
  Delay : Delay  Commented=on  DelayLength=round((td/1e-8)/2)
  MATLAB Function : MATLAB Function  TreatAsAtomicUnit=on
  Sum1 : Sum  Inputs=|-+
  Sum2 : Sum  Inputs=|++
  Variable Integer Delay : Delay  DelayLengthSource=Input port
      settings: InputPortMap=u0,p1
  Out1 : Outport
  wires:
  Variable Integer Delay/1 -> Sum1/2
  Sum1/1 -> Sum2/2
  Sum2/1 -> Out1/1
  In2/1 -> MATLAB Function/1(u), Sum2/1
  MATLAB Function/1(y) -> Sum1/1, Variable Integer Delay/1
  td/1 -> Variable Integer Delay/2
  delta/1 -> MATLAB Function/2(delta)

== system ICCMA_posicast_23_parallelGCNM_FO/posicast2 ==
  In2 : Inport
  delta : Inport  Port=2
  td : Inport  Port=3
  Delay : Delay  Commented=on  DelayLength=round((td/1e-8)/2)
  MATLAB Function : MATLAB Function  TreatAsAtomicUnit=on
  Sum1 : Sum  Inputs=|-+
  Sum2 : Sum  Inputs=|++
  Variable Integer Delay : Delay  DelayLengthSource=Input port
      settings: InputPortMap=u0,p1
  Out1 : Outport
  wires:
  Variable Integer Delay/1 -> Sum1/2
  Sum1/1 -> Sum2/2
  Sum2/1 -> Out1/1
  In2/1 -> MATLAB Function/1(u), Sum2/1
  MATLAB Function/1(y) -> Sum1/1, Variable Integer Delay/1
  td/1 -> Variable Integer Delay/2
  delta/1 -> MATLAB Function/2(delta)

== system ICCMA_posicast_23_parallelGCNM_FO/posicast3 ==
  In2 : Inport
  delta : Inport  Port=2
  td : Inport  Port=3
  Delay : Delay  Commented=on  DelayLength=round((td/1e-8)/2)
  MATLAB Function : MATLAB Function  TreatAsAtomicUnit=on
  Sum1 : Sum  Inputs=|-+
  Sum2 : Sum  Inputs=|++
  Variable Integer Delay : Delay  DelayLengthSource=Input port
      settings: InputPortMap=u0,p1
  Out1 : Outport
  wires:
  Variable Integer Delay/1 -> Sum1/2
  Sum1/1 -> Sum2/2
  Sum2/1 -> Out1/1
  In2/1 -> MATLAB Function/1(u), Sum2/1
  MATLAB Function/1(y) -> Sum1/1, Variable Integer Delay/1
  td/1 -> Variable Integer Delay/2
  delta/1 -> MATLAB Function/2(delta)

== system ICCMA_posicast_23_parallelGCNM_FO/posicast4 ==
  In2 : Inport
  delta : Inport  Port=2
  td : Inport  Port=3
  Delay : Delay  Commented=on  DelayLength=round((td/1e-8)/2)
  MATLAB Function : MATLAB Function  TreatAsAtomicUnit=on
  Sum1 : Sum  Inputs=|-+
  Sum2 : Sum  Inputs=|++
  Variable Integer Delay : Delay  DelayLengthSource=Input port
      settings: InputPortMap=u0,p1
  Out1 : Outport
  wires:
  Variable Integer Delay/1 -> Sum1/2
  Sum1/1 -> Sum2/2
  Sum2/1 -> Out1/1
  In2/1 -> MATLAB Function/1(u), Sum2/1
  MATLAB Function/1(y) -> Sum1/1, Variable Integer Delay/1
  td/1 -> Variable Integer Delay/2
  delta/1 -> MATLAB Function/2(delta)

== system ICCMA_posicast_23_parallelGCNM_FO/posicast5 ==
  In2 : Inport
  delta : Inport  Port=2
  td : Inport  Port=3
  Delay : Delay  Commented=on  DelayLength=round((td/1e-8)/2)
  MATLAB Function : MATLAB Function  TreatAsAtomicUnit=on
  Sum1 : Sum  Inputs=|-+
  Sum2 : Sum  Inputs=|++
  Variable Integer Delay : Delay  DelayLengthSource=Input port
      settings: InputPortMap=u0,p1
  Out1 : Outport
  wires:
  Variable Integer Delay/1 -> Sum1/2
  Sum1/1 -> Sum2/2
  Sum2/1 -> Out1/1
  In2/1 -> MATLAB Function/1(u), Sum2/1
  MATLAB Function/1(y) -> Sum1/1, Variable Integer Delay/1
  td/1 -> Variable Integer Delay/2
  delta/1 -> MATLAB Function/2(delta)

== system ICCMA_posicast_23_parallelGCNM_FO/posicast6 ==
  In2 : Inport
  delta : Inport  Port=2
  td : Inport  Port=3
  Delay : Delay  Commented=on  DelayLength=round((td/1e-8)/2)
  MATLAB Function : MATLAB Function  TreatAsAtomicUnit=on
  Sum1 : Sum  Inputs=|-+
  Sum2 : Sum  Inputs=|++
  Variable Integer Delay : Delay  DelayLengthSource=Input port
      settings: InputPortMap=u0,p1
  Out1 : Outport
  wires:
  Variable Integer Delay/1 -> Sum1/2
  Sum1/1 -> Sum2/2
  Sum2/1 -> Out1/1
  In2/1 -> MATLAB Function/1(u), Sum2/1
  MATLAB Function/1(y) -> Sum1/1, Variable Integer Delay/1
  td/1 -> Variable Integer Delay/2
  delta/1 -> MATLAB Function/2(delta)

== system ICCMA_posicast_23_parallelGCNM_FO/posicast7 ==
  In2 : Inport
  delta : Inport  Port=2
  td : Inport  Port=3
  Delay : Delay  Commented=on  DelayLength=round((td/1e-8)/2)
  MATLAB Function : MATLAB Function  TreatAsAtomicUnit=on
  Sum1 : Sum  Inputs=|-+
  Sum2 : Sum  Inputs=|++
  Variable Integer Delay : Delay  DelayLengthSource=Input port
      settings: InputPortMap=u0,p1
  Out1 : Outport
  wires:
  Variable Integer Delay/1 -> Sum1/2
  Sum1/1 -> Sum2/2
  Sum2/1 -> Out1/1
  In2/1 -> MATLAB Function/1(u), Sum2/1
  MATLAB Function/1(y) -> Sum1/1, Variable Integer Delay/1
  td/1 -> Variable Integer Delay/2
  delta/1 -> MATLAB Function/2(delta)

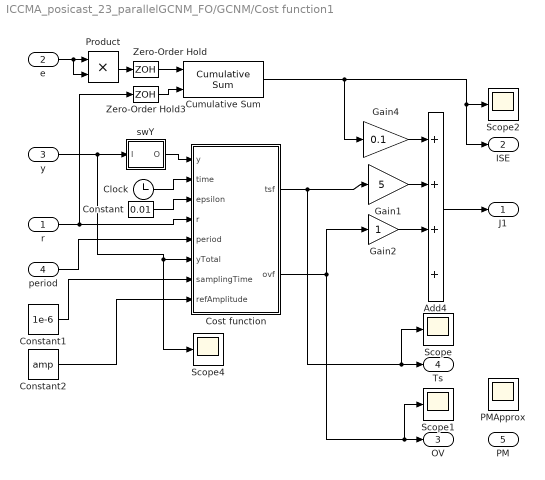
== system ICCMA_posicast_23_parallelGCNM_FO/GCNM/Cost function1 ==
  r : Inport
  e : Inport  Port=2
  y : Inport  Port=3
  period : Inport  Port=4
  Add4 : Sum  Inputs=++++
  Clock : Clock
  Constant : Constant  Value=0.01
  Constant1 : Constant  Value=1e-6
  Constant2 : Constant  Value=amp
  Cost function : MATLAB Function  TreatAsAtomicUnit=on
  Cumulative Sum : dspmathops/Cumulative Sum  dim=Channels (running sum)  InputProcessing=Columns as channels (frame based)  reset_popup=Falling edge  roundingMode=Floor  overflowMode=off  outputDataTypeStr=Inherit: Same as accumulator  outputMin=[]  outputMax=[]  outputLastDataTypeStr=Inherit: Same as accumulator
  Gain1 : Gain  Gain=5
  Gain2 : Gain
  Gain4 : Gain  Gain=0.1
  PMApprox : Scope
  Product : Product
  Scope{,1..2,4} (4 alike) : Scope
  Zero-Order Hold : ZeroOrderHold  SampleTime=-1
  Zero-Order Hold3 : ZeroOrderHold  SampleTime=-1
  swY : Subsystem
  J1 : Outport
  ISE : Outport  Port=2
  OV : Outport  Port=3
  Ts : Outport  Port=4
  PM : Outport  Port=5
  wires:
  Constant2/1 -> Cost function/8(refAmplitude)
  Gain4/1 -> Add4/1
  Cost function/2(ovf) -> OV/1, Scope1/1, Gain2/1
  Cost function/1(tsf) -> Ts/1, Scope/1, Gain1/1
  Gain1/1 -> Add4/2
  Constant1/1 -> Cost function/7(samplingTime)
  period/1 -> Cost function/5(period)
  Gain2/1 -> Add4/3
  Add4/1 -> J1/1
  y/1 -> swY/1(I), Cost function/6(yTotal), Scope4/1
  Constant/1 -> Cost function/3(epsilon)
  Product/1 -> Zero-Order Hold/1
  Clock/1 -> Cost function/2(time)
  swY/1(O) -> Cost function/1(y)
  r/1 -> Cost function/4(r), Zero-Order Hold3/1
  Zero-Order Hold/1 -> Cumulative Sum/1
  e/1 -> Product/1, Product/2
  Zero-Order Hold3/1 -> Cumulative Sum/2
  Cumulative Sum/1 -> Scope2/1, ISE/1, Gain4/1

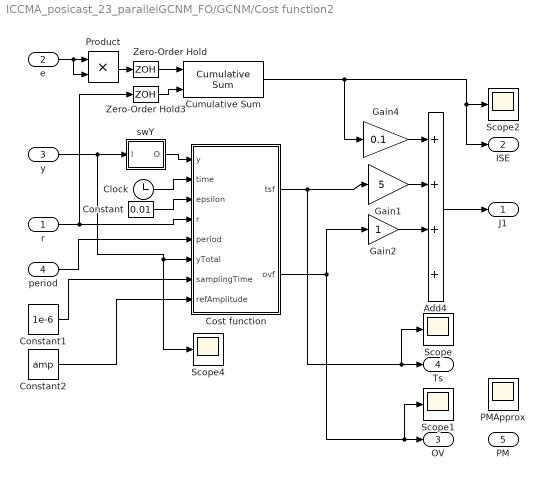
== system ICCMA_posicast_23_parallelGCNM_FO/GCNM/Cost function2 ==
  r : Inport
  e : Inport  Port=2
  y : Inport  Port=3
  period : Inport  Port=4
  Add4 : Sum  Inputs=++++
  Clock : Clock
  Constant : Constant  Value=0.01
  Constant1 : Constant  Value=1e-6
  Constant2 : Constant  Value=amp
  Cost function : MATLAB Function  TreatAsAtomicUnit=on
  Cumulative Sum : dspmathops/Cumulative Sum  dim=Channels (running sum)  InputProcessing=Columns as channels (frame based)  reset_popup=Falling edge  roundingMode=Floor  overflowMode=off  outputDataTypeStr=Inherit: Same as accumulator  outputMin=[]  outputMax=[]  outputLastDataTypeStr=Inherit: Same as accumulator
  Gain1 : Gain  Gain=5
  Gain2 : Gain
  Gain4 : Gain  Gain=0.1
  PMApprox : Scope
  Product : Product
  Scope{,1..2,4} (4 alike) : Scope
  Zero-Order Hold : ZeroOrderHold  SampleTime=-1
  Zero-Order Hold3 : ZeroOrderHold  SampleTime=-1
  swY : Subsystem
  J1 : Outport
  ISE : Outport  Port=2
  OV : Outport  Port=3
  Ts : Outport  Port=4
  PM : Outport  Port=5
  wires:
  Cumulative Sum/1 -> Gain4/1, ISE/1, Scope2/1
  Zero-Order Hold3/1 -> Cumulative Sum/2
  e/1 -> Product/2, Product/1
  Zero-Order Hold/1 -> Cumulative Sum/1
  r/1 -> Zero-Order Hold3/1, Cost function/4(r)
  swY/1(O) -> Cost function/1(y)
  Clock/1 -> Cost function/2(time)
  Product/1 -> Zero-Order Hold/1
  Constant/1 -> Cost function/3(epsilon)
  y/1 -> Scope4/1, Cost function/6(yTotal), swY/1(I)
  Add4/1 -> J1/1
  Gain2/1 -> Add4/3
  period/1 -> Cost function/5(period)
  Constant1/1 -> Cost function/7(samplingTime)
  Gain1/1 -> Add4/2
  Cost function/1(tsf) -> Gain1/1, Scope/1, Ts/1
  Cost function/2(ovf) -> Gain2/1, Scope1/1, OV/1
  Gain4/1 -> Add4/1
  Constant2/1 -> Cost function/8(refAmplitude)

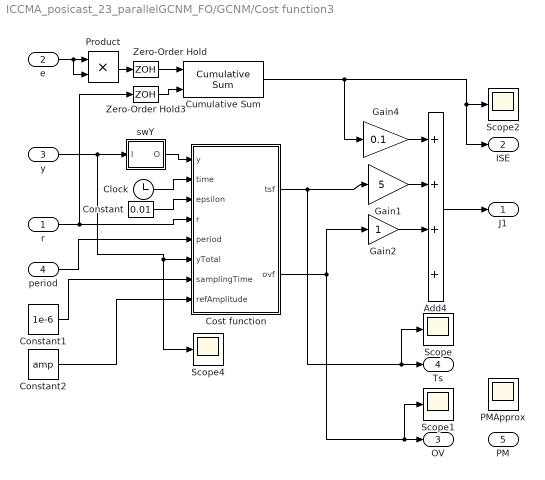
== system ICCMA_posicast_23_parallelGCNM_FO/GCNM/Cost function3 ==
  r : Inport
  e : Inport  Port=2
  y : Inport  Port=3
  period : Inport  Port=4
  Add4 : Sum  Inputs=++++
  Clock : Clock
  Constant : Constant  Value=0.01
  Constant1 : Constant  Value=1e-6
  Constant2 : Constant  Value=amp
  Cost function : MATLAB Function  TreatAsAtomicUnit=on
  Cumulative Sum : dspmathops/Cumulative Sum  dim=Channels (running sum)  InputProcessing=Columns as channels (frame based)  reset_popup=Falling edge  roundingMode=Floor  overflowMode=off  outputDataTypeStr=Inherit: Same as accumulator  outputMin=[]  outputMax=[]  outputLastDataTypeStr=Inherit: Same as accumulator
  Gain1 : Gain  Gain=5
  Gain2 : Gain
  Gain4 : Gain  Gain=0.1
  PMApprox : Scope
  Product : Product
  Scope{,1..2,4} (4 alike) : Scope
  Zero-Order Hold : ZeroOrderHold  SampleTime=-1
  Zero-Order Hold3 : ZeroOrderHold  SampleTime=-1
  swY : Subsystem
  J1 : Outport
  ISE : Outport  Port=2
  OV : Outport  Port=3
  Ts : Outport  Port=4
  PM : Outport  Port=5
  wires:
  Cumulative Sum/1 -> Gain4/1, ISE/1, Scope2/1
  Zero-Order Hold3/1 -> Cumulative Sum/2
  e/1 -> Product/2, Product/1
  Zero-Order Hold/1 -> Cumulative Sum/1
  r/1 -> Zero-Order Hold3/1, Cost function/4(r)
  swY/1(O) -> Cost function/1(y)
  Clock/1 -> Cost function/2(time)
  Product/1 -> Zero-Order Hold/1
  Constant/1 -> Cost function/3(epsilon)
  y/1 -> Scope4/1, Cost function/6(yTotal), swY/1(I)
  Add4/1 -> J1/1
  Gain2/1 -> Add4/3
  period/1 -> Cost function/5(period)
  Constant1/1 -> Cost function/7(samplingTime)
  Gain1/1 -> Add4/2
  Cost function/1(tsf) -> Gain1/1, Scope/1, Ts/1
  Cost function/2(ovf) -> Gain2/1, Scope1/1, OV/1
  Gain4/1 -> Add4/1
  Constant2/1 -> Cost function/8(refAmplitude)

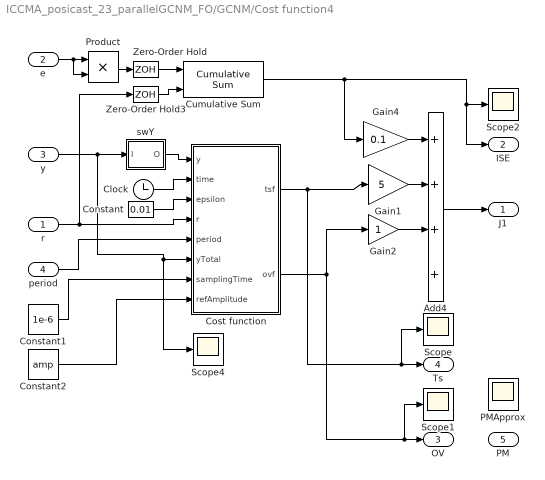
== system ICCMA_posicast_23_parallelGCNM_FO/GCNM/Cost function4 ==
  r : Inport
  e : Inport  Port=2
  y : Inport  Port=3
  period : Inport  Port=4
  Add4 : Sum  Inputs=++++
  Clock : Clock
  Constant : Constant  Value=0.01
  Constant1 : Constant  Value=1e-6
  Constant2 : Constant  Value=amp
  Cost function : MATLAB Function  TreatAsAtomicUnit=on
  Cumulative Sum : dspmathops/Cumulative Sum  dim=Channels (running sum)  InputProcessing=Columns as channels (frame based)  reset_popup=Falling edge  roundingMode=Floor  overflowMode=off  outputDataTypeStr=Inherit: Same as accumulator  outputMin=[]  outputMax=[]  outputLastDataTypeStr=Inherit: Same as accumulator
  Gain1 : Gain  Gain=5
  Gain2 : Gain
  Gain4 : Gain  Gain=0.1
  PMApprox : Scope
  Product : Product
  Scope{,1..2,4} (4 alike) : Scope
  Zero-Order Hold : ZeroOrderHold  SampleTime=-1
  Zero-Order Hold3 : ZeroOrderHold  SampleTime=-1
  swY : Subsystem
  J1 : Outport
  ISE : Outport  Port=2
  OV : Outport  Port=3
  Ts : Outport  Port=4
  PM : Outport  Port=5
  wires:
  Constant2/1 -> Cost function/8(refAmplitude)
  Gain4/1 -> Add4/1
  Cost function/2(ovf) -> OV/1, Scope1/1, Gain2/1
  Cost function/1(tsf) -> Ts/1, Scope/1, Gain1/1
  Gain1/1 -> Add4/2
  Constant1/1 -> Cost function/7(samplingTime)
  period/1 -> Cost function/5(period)
  Gain2/1 -> Add4/3
  Add4/1 -> J1/1
  y/1 -> swY/1(I), Cost function/6(yTotal), Scope4/1
  Constant/1 -> Cost function/3(epsilon)
  Product/1 -> Zero-Order Hold/1
  Clock/1 -> Cost function/2(time)
  swY/1(O) -> Cost function/1(y)
  r/1 -> Cost function/4(r), Zero-Order Hold3/1
  Zero-Order Hold/1 -> Cumulative Sum/1
  e/1 -> Product/1, Product/2
  Zero-Order Hold3/1 -> Cumulative Sum/2
  Cumulative Sum/1 -> Scope2/1, ISE/1, Gain4/1

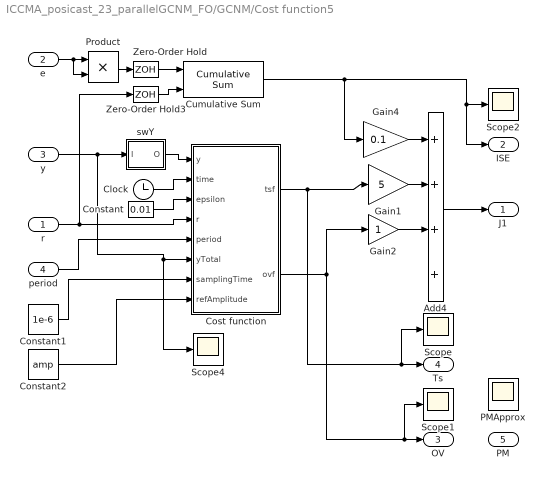
== system ICCMA_posicast_23_parallelGCNM_FO/GCNM/Cost function5 ==
  r : Inport
  e : Inport  Port=2
  y : Inport  Port=3
  period : Inport  Port=4
  Add4 : Sum  Inputs=++++
  Clock : Clock
  Constant : Constant  Value=0.01
  Constant1 : Constant  Value=1e-6
  Constant2 : Constant  Value=amp
  Cost function : MATLAB Function  TreatAsAtomicUnit=on
  Cumulative Sum : dspmathops/Cumulative Sum  dim=Channels (running sum)  InputProcessing=Columns as channels (frame based)  reset_popup=Falling edge  roundingMode=Floor  overflowMode=off  outputDataTypeStr=Inherit: Same as accumulator  outputMin=[]  outputMax=[]  outputLastDataTypeStr=Inherit: Same as accumulator
  Gain1 : Gain  Gain=5
  Gain2 : Gain
  Gain4 : Gain  Gain=0.1
  PMApprox : Scope
  Product : Product
  Scope{,1..2,4} (4 alike) : Scope
  Zero-Order Hold : ZeroOrderHold  SampleTime=-1
  Zero-Order Hold3 : ZeroOrderHold  SampleTime=-1
  swY : Subsystem
  J1 : Outport
  ISE : Outport  Port=2
  OV : Outport  Port=3
  Ts : Outport  Port=4
  PM : Outport  Port=5
  wires:
  Constant2/1 -> Cost function/8(refAmplitude)
  Gain4/1 -> Add4/1
  Cost function/2(ovf) -> OV/1, Scope1/1, Gain2/1
  Cost function/1(tsf) -> Ts/1, Scope/1, Gain1/1
  Gain1/1 -> Add4/2
  Constant1/1 -> Cost function/7(samplingTime)
  period/1 -> Cost function/5(period)
  Gain2/1 -> Add4/3
  Add4/1 -> J1/1
  y/1 -> swY/1(I), Cost function/6(yTotal), Scope4/1
  Constant/1 -> Cost function/3(epsilon)
  Product/1 -> Zero-Order Hold/1
  Clock/1 -> Cost function/2(time)
  swY/1(O) -> Cost function/1(y)
  r/1 -> Cost function/4(r), Zero-Order Hold3/1
  Zero-Order Hold/1 -> Cumulative Sum/1
  e/1 -> Product/1, Product/2
  Zero-Order Hold3/1 -> Cumulative Sum/2
  Cumulative Sum/1 -> Scope2/1, ISE/1, Gain4/1

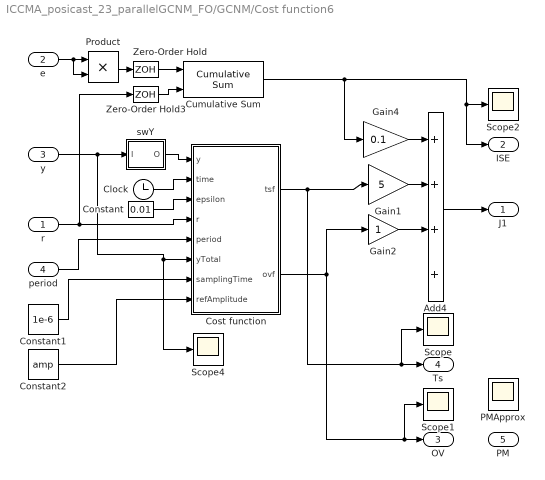
== system ICCMA_posicast_23_parallelGCNM_FO/GCNM/Cost function6 ==
  r : Inport
  e : Inport  Port=2
  y : Inport  Port=3
  period : Inport  Port=4
  Add4 : Sum  Inputs=++++
  Clock : Clock
  Constant : Constant  Value=0.01
  Constant1 : Constant  Value=1e-6
  Constant2 : Constant  Value=amp
  Cost function : MATLAB Function  TreatAsAtomicUnit=on
  Cumulative Sum : dspmathops/Cumulative Sum  dim=Channels (running sum)  InputProcessing=Columns as channels (frame based)  reset_popup=Falling edge  roundingMode=Floor  overflowMode=off  outputDataTypeStr=Inherit: Same as accumulator  outputMin=[]  outputMax=[]  outputLastDataTypeStr=Inherit: Same as accumulator
  Gain1 : Gain  Gain=5
  Gain2 : Gain
  Gain4 : Gain  Gain=0.1
  PMApprox : Scope
  Product : Product
  Scope{,1..2,4} (4 alike) : Scope
  Zero-Order Hold : ZeroOrderHold  SampleTime=-1
  Zero-Order Hold3 : ZeroOrderHold  SampleTime=-1
  swY : Subsystem
  J1 : Outport
  ISE : Outport  Port=2
  OV : Outport  Port=3
  Ts : Outport  Port=4
  PM : Outport  Port=5
  wires:
  Cumulative Sum/1 -> Gain4/1, ISE/1, Scope2/1
  Zero-Order Hold3/1 -> Cumulative Sum/2
  e/1 -> Product/2, Product/1
  Zero-Order Hold/1 -> Cumulative Sum/1
  r/1 -> Zero-Order Hold3/1, Cost function/4(r)
  swY/1(O) -> Cost function/1(y)
  Clock/1 -> Cost function/2(time)
  Product/1 -> Zero-Order Hold/1
  Constant/1 -> Cost function/3(epsilon)
  y/1 -> Scope4/1, Cost function/6(yTotal), swY/1(I)
  Add4/1 -> J1/1
  Gain2/1 -> Add4/3
  period/1 -> Cost function/5(period)
  Constant1/1 -> Cost function/7(samplingTime)
  Gain1/1 -> Add4/2
  Cost function/1(tsf) -> Gain1/1, Scope/1, Ts/1
  Cost function/2(ovf) -> Gain2/1, Scope1/1, OV/1
  Gain4/1 -> Add4/1
  Constant2/1 -> Cost function/8(refAmplitude)

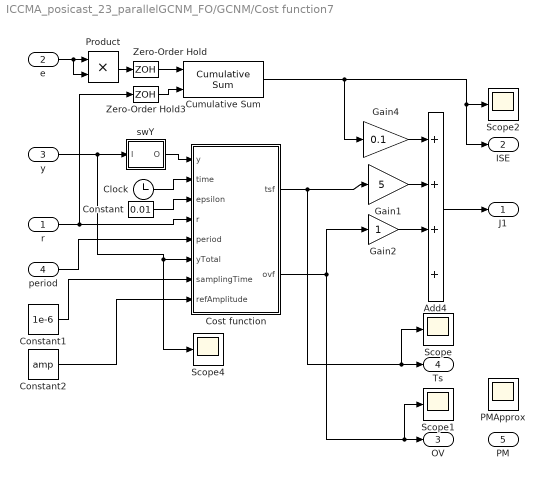
== system ICCMA_posicast_23_parallelGCNM_FO/GCNM/Cost function7 ==
  r : Inport
  e : Inport  Port=2
  y : Inport  Port=3
  period : Inport  Port=4
  Add4 : Sum  Inputs=++++
  Clock : Clock
  Constant : Constant  Value=0.01
  Constant1 : Constant  Value=1e-6
  Constant2 : Constant  Value=amp
  Cost function : MATLAB Function  TreatAsAtomicUnit=on
  Cumulative Sum : dspmathops/Cumulative Sum  dim=Channels (running sum)  InputProcessing=Columns as channels (frame based)  reset_popup=Falling edge  roundingMode=Floor  overflowMode=off  outputDataTypeStr=Inherit: Same as accumulator  outputMin=[]  outputMax=[]  outputLastDataTypeStr=Inherit: Same as accumulator
  Gain1 : Gain  Gain=5
  Gain2 : Gain
  Gain4 : Gain  Gain=0.1
  PMApprox : Scope
  Product : Product
  Scope{,1..2,4} (4 alike) : Scope
  Zero-Order Hold : ZeroOrderHold  SampleTime=-1
  Zero-Order Hold3 : ZeroOrderHold  SampleTime=-1
  swY : Subsystem
  J1 : Outport
  ISE : Outport  Port=2
  OV : Outport  Port=3
  Ts : Outport  Port=4
  PM : Outport  Port=5
  wires:
  Cumulative Sum/1 -> Gain4/1, ISE/1, Scope2/1
  Zero-Order Hold3/1 -> Cumulative Sum/2
  e/1 -> Product/2, Product/1
  Zero-Order Hold/1 -> Cumulative Sum/1
  r/1 -> Zero-Order Hold3/1, Cost function/4(r)
  swY/1(O) -> Cost function/1(y)
  Clock/1 -> Cost function/2(time)
  Product/1 -> Zero-Order Hold/1
  Constant/1 -> Cost function/3(epsilon)
  y/1 -> Scope4/1, Cost function/6(yTotal), swY/1(I)
  Add4/1 -> J1/1
  Gain2/1 -> Add4/3
  period/1 -> Cost function/5(period)
  Constant1/1 -> Cost function/7(samplingTime)
  Gain1/1 -> Add4/2
  Cost function/1(tsf) -> Gain1/1, Scope/1, Ts/1
  Cost function/2(ovf) -> Gain2/1, Scope1/1, OV/1
  Gain4/1 -> Add4/1
  Constant2/1 -> Cost function/8(refAmplitude)

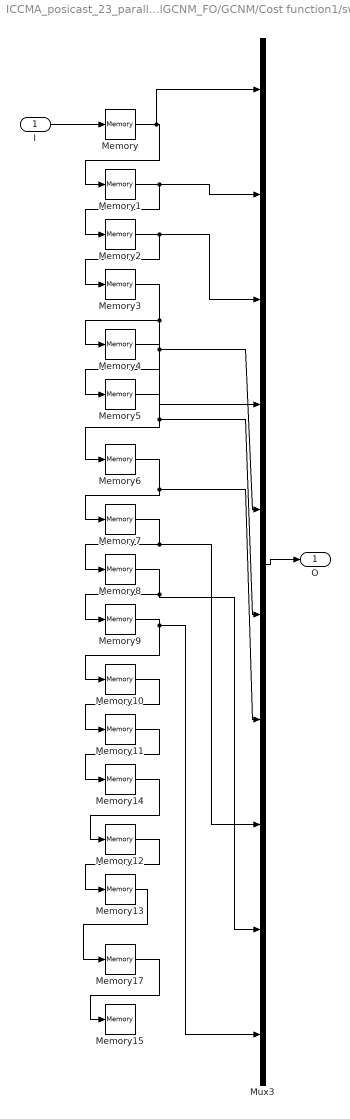
== system ICCMA_posicast_23_parallelGCNM_FO/GCNM/Cost function1/swY ==
  I : Inport
  Memory{,1..15,17} (17 alike) : Memory
  Mux3 : Mux  Inputs=10
  O : Outport
  wires:
  Memory17/1 -> Memory15/1
  Memory7/1 -> Mux3/8, Memory8/1
  Memory/1 -> Mux3/1, Memory1/1
  Memory8/1 -> Mux3/9, Memory9/1
  I/1 -> Memory/1
  Memory2/1 -> Mux3/3, Memory3/1
  Memory10/1 -> Memory11/1
  Memory1/1 -> Mux3/2, Memory2/1
  Memory6/1 -> Mux3/7, Memory7/1
  Memory3/1 -> Mux3/4, Memory4/1
  Memory9/1 -> Mux3/10, Memory10/1
  Mux3/1 -> O/1
  Memory4/1 -> Mux3/5, Memory5/1
  Memory5/1 -> Mux3/6, Memory6/1
  Memory13/1 -> Memory17/1
  Memory12/1 -> Memory13/1
  Memory14/1 -> Memory12/1
  Memory11/1 -> Memory14/1

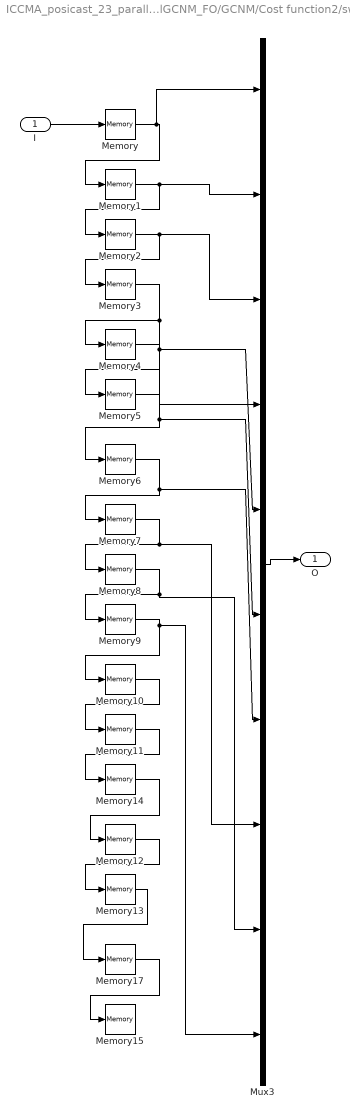
== system ICCMA_posicast_23_parallelGCNM_FO/GCNM/Cost function2/swY ==
  I : Inport
  Memory{,1..15,17} (17 alike) : Memory
  Mux3 : Mux  Inputs=10
  O : Outport
  wires:
  Memory11/1 -> Memory14/1
  Memory14/1 -> Memory12/1
  Memory12/1 -> Memory13/1
  Memory13/1 -> Memory17/1
  Memory5/1 -> Memory6/1, Mux3/6
  Memory4/1 -> Memory5/1, Mux3/5
  Mux3/1 -> O/1
  Memory9/1 -> Memory10/1, Mux3/10
  Memory3/1 -> Memory4/1, Mux3/4
  Memory6/1 -> Memory7/1, Mux3/7
  Memory1/1 -> Memory2/1, Mux3/2
  Memory10/1 -> Memory11/1
  Memory2/1 -> Memory3/1, Mux3/3
  I/1 -> Memory/1
  Memory8/1 -> Memory9/1, Mux3/9
  Memory/1 -> Memory1/1, Mux3/1
  Memory7/1 -> Memory8/1, Mux3/8
  Memory17/1 -> Memory15/1

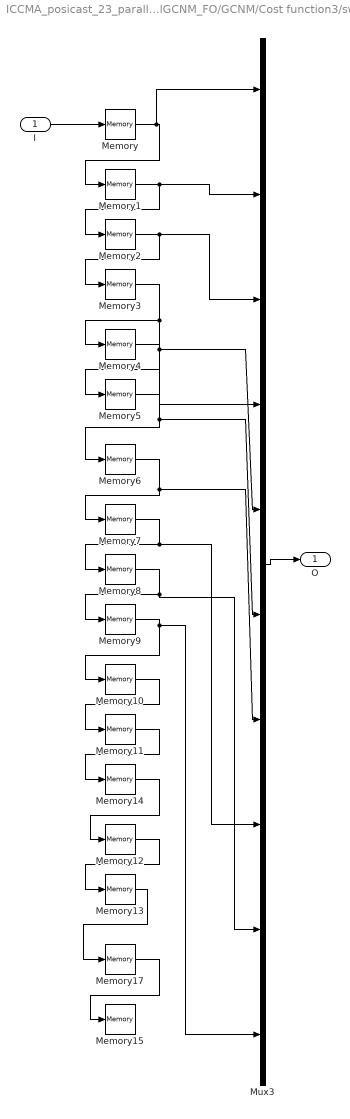
== system ICCMA_posicast_23_parallelGCNM_FO/GCNM/Cost function3/swY ==
  I : Inport
  Memory{,1..15,17} (17 alike) : Memory
  Mux3 : Mux  Inputs=10
  O : Outport
  wires:
  Memory11/1 -> Memory14/1
  Memory14/1 -> Memory12/1
  Memory12/1 -> Memory13/1
  Memory13/1 -> Memory17/1
  Memory5/1 -> Memory6/1, Mux3/6
  Memory4/1 -> Memory5/1, Mux3/5
  Mux3/1 -> O/1
  Memory9/1 -> Memory10/1, Mux3/10
  Memory3/1 -> Memory4/1, Mux3/4
  Memory6/1 -> Memory7/1, Mux3/7
  Memory1/1 -> Memory2/1, Mux3/2
  Memory10/1 -> Memory11/1
  Memory2/1 -> Memory3/1, Mux3/3
  I/1 -> Memory/1
  Memory8/1 -> Memory9/1, Mux3/9
  Memory/1 -> Memory1/1, Mux3/1
  Memory7/1 -> Memory8/1, Mux3/8
  Memory17/1 -> Memory15/1
